simulink model "StopWatch2_2018a"  (R2018a)
settings: Solver=VariableStepDiscrete  StartTime=0.0  StopTime=1  MaxStep=0.1  RelTol=1e-3
settings Model: Creator=86188  LastModifiedBy=bzhan

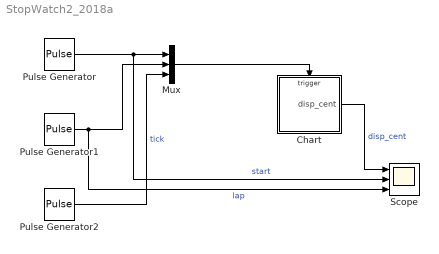
== system StopWatch2_2018a ==
  Chart : Stateflow chart  TreatAsAtomicUnit=on
  Mux : Mux  Inputs=3
  Pulse Generator : DiscretePulseGenerator  PulseType=Time based  Period=0.3  PulseWidth=30  PhaseDelay=0.03
  Pulse Generator1 : DiscretePulseGenerator  PulseType=Time based  Period=0.1  PulseWidth=30  PhaseDelay=0.05
  Pulse Generator2 : DiscretePulseGenerator  PulseType=Time based  Period=0.01  PulseWidth=50
  Scope : Scope  NumInputPorts=3
  wires:
  Pulse Generator/1 -> Scope/2, Mux/1  "start"
  Pulse Generator1/1 -> Scope/3, Mux/2  "lap"
  Mux/1 -> Chart/Trigger
  Pulse Generator2/1 -> Mux/3  "tick"
  Chart/1(disp_cent) -> Scope/1  "disp_cent"

== stateflow chart StopWatch2_2018a/Chart ==
  settings: executeAtInitialization=1
  state StopW
    en:f("en_StopW")
    state Reset
      en:f("Reset")
      Reset -> (junction 5) [order 1] : LAP{cent=0;sec=0;
          | mins=0;disp_cent=0;
          | disp_sec=0;disp_min=0;}
    state LapStop
      en:f("LapStop")
    (default) -> Reset
    LapStop -> Reset [order 2] : LAP
  state RunW
    state Running
      en:f("Running")
      during:
      disp_cent=cent;
      disp_sec=sec;
      disp_min=mins;
    state Lap
      en:f("Lap")
    RunW -> (junction 19) : TIC{cent=cent+1;}
    (junction 19) -> (junction 25) [order 2]
    (junction 19) -> (junction 21) [order 1] : [cent==100]{cent=0;sec=sec+1;}
    (junction 21) -> (junction 25) [order 2]
    (junction 21) -> (junction 25) [order 1] : [sec==60]{sec=0;mins=mins+1;}
    Running -> Lap [order 2] : LAP
    Lap -> Running [order 2] : LAP
  (default) -> StopW
  Reset -> Running [order 1] : START
  Running -> Reset [order 1] : START
  LapStop -> Lap [order 1] : START
  Lap -> LapStop [order 1] : START
  data: s function_input; cent local =0; mins local =0; disp_min local; sec local =0; disp_sec local =0; disp_cent output
  events: START input RISING_EDGE_EVENT; LAP input RISING_EDGE_EVENT; TIC input RISING_EDGE_EVENT
  function f(s):
    | function f(s)
    |     fprintf(s+"\n");
